simulink model "et_robocon_dev_guy"  (R2013b)
settings: Solver=FixedStepDiscrete  SolverMode=SingleTasking  StartTime=0.0  StopTime=inf  FixedStep=balancer_ts  RelTol=1e-3
undefined symbols (not defined in the file): a_d, a_r, balancerStates_Bus0, Batt, battery_gain, battery_offset, cmd_max, current_mode_status, current_task_operation_status, DiscIntNeverNeededParam, exec_period, Init_Bus0, k_f, k_i, k_phidot, k_thetadot, lightCalib, R, STATE, TRACK_MODE_LIST, ts2, W
libraries: simulink x29, legonxtlib x28, simulink_extras x4, light_sensor_calibration_algorithm_atomic_sub_chart_library x3, gyro_calibration_algorithm_atomic_sub_chart_library x1, limbo_algorithm_atomic_sub_chart_library x1, see_saw x1
(part 2 of 3)

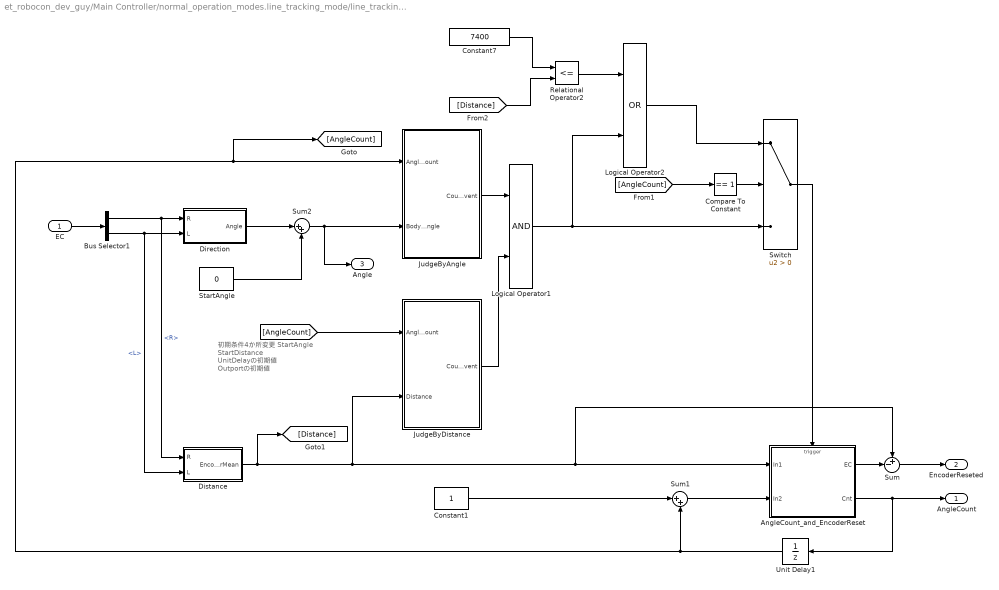
== system et_robocon_dev_guy/Main Controller/normal_operation_modes.line_tracking_mode/line_tracking_mode.processLight/LineTracePID/AngleCounter ==
  note: 初期条件4か所変更
      | StartAngle
      | StartDistance
      | UnitDelayの初期値
      | Outportの初期値
  EC : Inport
  AngleCount_and_EncoderReset : Subsystem  TreatAsAtomicUnit=on
  Bus Selector1 : BusSelector  OutputSignals=R,L
  Compare To Constant : simulink/Logic and Bit Operations/Compare To Constant  relop===  const=1  OutDataTypeStr=boolean
  Constant1 : Constant  OutDataTypeStr=uint8
  Constant7 : Constant  Value=7400  OutDataTypeStr=int32
  Direction : Subsystem
  Distance : Subsystem
  JudgeByAngle : Subsystem
  JudgeByDistance : Subsystem
  Logical Operator1 : Logic  AllPortsSameDT=off  OutDataTypeStr=boolean
  Logical Operator2 : Logic  Operator=OR  AllPortsSameDT=off  OutDataTypeStr=boolean
  Relational Operator2 : RelationalOperator  Operator=<=  OutDataTypeStr=boolean
  StartAngle : Constant  Value=0  OutDataTypeStr=int16
  Sum : Sum  Inputs=+-|
  Sum1 : Sum  Inputs=|++  AccumDataTypeStr=uint8
  Sum2 : Sum  Inputs=|++
  Switch : Switch  Criteria=u2 > Threshold
  Unit Delay1 : UnitDelay  InitialCondition=1  SampleTime=-1
  AngleCount : Outport
  EncoderReseted : Outport  Port=2
  Angle : Outport  Port=3
  wires:
  Sum2/1 -> JudgeByAngle/2(BodyAngle), Angle/1
  Sum1/1 -> AngleCount_and_EncoderReset/2(In2)
  Constant1/1 -> Sum1/1
  Unit Delay1/1 -> [AngleCount], JudgeByAngle/1(AngleCount), Sum1/2
  AngleCount_and_EncoderReset/2(Cnt) -> AngleCount/1, Unit Delay1/1
  Bus Selector1/1 -> Distance/1(R), Direction/1(R)  "<R>"
  Bus Selector1/2 -> Distance/2(L), Direction/2(L)  "<L>"
  EC/1 -> Bus Selector1/1
  AngleCount_and_EncoderReset/1(EC) -> Sum/2
  Sum/1 -> EncoderReseted/1
  Distance/1(EncoderMean) -> [Distance], JudgeByDistance/2(Distance), Sum/1, AngleCount_and_EncoderReset/1(In1)
  [AngleCount] -> JudgeByDistance/1(AngleCount)
  JudgeByAngle/1(CountEvent) -> Logical Operator1/1
  JudgeByDistance/1(CountEvent) -> Logical Operator1/2
  Direction/1(Angle) -> Sum2/1
  StartAngle/1 -> Sum2/2
  Logical Operator1/1 -> Logical Operator2/2, Switch/3
  Switch/1 -> AngleCount_and_EncoderReset/Trigger
  Compare To Constant/1 -> Switch/2
  [AngleCount] -> Compare To Constant/1
  Logical Operator2/1 -> Switch/1
  Constant7/1 -> Relational Operator2/1
  Relational Operator2/1 -> Logical Operator2/1
  [Distance] -> Relational Operator2/2

== system et_robocon_dev_guy/Main Controller/normal_operation_modes.line_tracking_mode/line_tracking_mode.processLight/LineTracePID/Handler ==
  steering : Inport
  fwd : Inport  Port=2
  sw : Inport  Port=3
  Constant1 : Constant  Value=-1  OutDataTypeStr=int8
  Lookup Table : Lookup  InputValues="[-30  -5  0  5 30]"  Table=[0.65 1 1 1 0.65]  RndMeth=Simplest
  Mux : Mux  Inputs=2
  Product : Product  OutDataTypeStr=single  RndMeth=Simplest
  Switch : Switch  OutDataTypeStr=single  RndMeth=Simplest
  Switch1 : Switch  OutDataTypeStr=single  RndMeth=Simplest
  rocket_start : Subsystem
  slow_start : Subsystem
  Out1 : Outport
  wires:
  Lookup Table/1 -> Product/2
  Product/1 -> Switch/3
  fwd/1 -> Switch/1, Product/1
  steering/1 -> Lookup Table/1, Mux/2  "str"
  sw/1 -> Switch/2
  slow_start/1(fwd_slow) -> Switch1/1
  Mux/1 -> Out1/1
  Switch/1 -> rocket_start/1(fwd), slow_start/1(fwd)  "fwd"
  Constant1/1 -> Switch1/2
  rocket_start/1(fwd_slow) -> Switch1/3
  Switch1/1 -> Mux/1

== system et_robocon_dev_guy/Main Controller/normal_operation_modes.line_tracking_mode/line_tracking_mode.processLight/LineTracePID/SwitchController ==
  Cnt : Inport
  EC_reseted : Inport  Port=2
  Angle : Inport  Port=3
  LigthSens : Inport  Port=4
  Gyro : Inport  Port=5
  BasicStage : Subsystem
  BonusStage : Subsystem
  Merge : Merge
  Merge1 : Merge
  Merge2 : Merge
  Flag_steering : Outport
  PID : Outport  Port=2
  fwd : Outport  Port=3
  bias : Outport  Port=4
  wires:
  Cnt/1 -> BonusStage/1(AngleCnt), BasicStage/1(AngleCnt)
  Merge/1 -> PID/1
  Merge1/1 -> fwd/1
  BasicStage/2(fwd) -> [fwd_Basic]
  [fwd_Basic] -> Merge1/1
  [fwd_Bonus] -> Merge1/2
  BasicStage/4(bias) -> [bias_Basic]
  [bias_Basic] -> Merge2/1
  [bias_Bonus] -> Merge2/2
  Merge2/1 -> bias/1
  EC_reseted/1 -> BasicStage/2(EC_reseted), BonusStage/2(EC_reseted)
  LigthSens/1 -> BonusStage/4(LightSens), BasicStage/4(LightSens)
  BasicStage/1(PID) -> Merge/1
  Gyro/1 -> BonusStage/3(Gyro)
  BonusStage/1(PID) -> Merge/2
  BonusStage/2(fwd) -> [fwd_Bonus]
  BonusStage/3(bias) -> [bias_Bonus]
  Angle/1 -> BasicStage/3(Angle)
  BasicStage/3(Flag_steering) -> Flag_steering/1

== system et_robocon_dev_guy/Main Controller/normal_operation_modes.line_tracking_mode/line_tracking_mode.processLight/LineTracePID/SwutchForFreeSteering ==
  note: Edge Change
      | -1: Run right edge
      | 1: Run left edge
  note: Target Value
  FlagSteering : Inport
  PID : Inport  Port=2
  LightSens : Inport  Port=3
  Add : Sum  Inputs=+-  AccumDataTypeStr=single  OutDataTypeStr=single  RndMeth=Simplest
  AdjustForUnit : Gain  Gain=18.25  OutDataTypeStr=single  RndMeth=Simplest
  Constant2 : Constant  OutDataTypeStr=single  SampleTime=-1
  Constant6 : Constant  Value=0.5  OutDataTypeStr=single  SampleTime=-1
  DeleteDummyData : Selector  InputPortWidth=5  IndexOptions=Index vector (dialog)  Indices=1  OutputSizes=1
  Product1 : Product  OutDataTypeStr=single  RndMeth=Simplest
  Switch : Switch  Criteria=u2 > Threshold
  tmpController : Subsystem  TreatAsAtomicUnit=on  mask(tmp PID Controller){Ts_=ts2, SaturationMax=100, SaturationMin=-100}
      mask prompts: Ts_ "Sampling Time (Task Period)"; SaturationMax "Saturation Max Value of PID Ctrl"; SaturationMin "Saturation Min Value of PID"
      mask help:
      | Sampling Time: Task Period
      | P: Proportional Gain
      | I: Integral Gain
      | D: Derivative Gain
      | B: Back Gain for Integrator
      | Saturation Max Value of PID ctrl:
      |    Saturation Max Value of PID ctrl > Saturation Min Value of PID ctrl
      | Saturation Min Value of PID ctrl:
      |    Saturation Min Value of PID ctrl < Saturation Max Value of PID ctrl
      settings: RTWSystemCode=Inline
      mask Display: disp('PID')
  Steering : Outport
  wires:
  PID/1 -> tmpController/2(BD), DeleteDummyData/1
  Switch/1 -> Steering/1
  DeleteDummyData/1 -> Switch/1  "FreeSteering"
  FlagSteering/1 -> Switch/2
  Add/1 -> Product1/1
  LightSens/1 -> Add/1
  Constant6/1 -> Add/2
  Constant2/1 -> Product1/2
  Product1/1 -> tmpController/1(Error)  "Diff_Between_Target_and_Value"
  tmpController/1(Target_deg) -> AdjustForUnit/1
  AdjustForUnit/1 -> Switch/3  "LintTraceSteering"

== system et_robocon_dev_guy/State Estimation/Data Type Conversion Unit Conversion Tail Initialization/Low Pass Filter/Store Offset ==
  x : Inport
  Enable : EnablePort
  x0 : Outport  InitialOutput=0
  wires:
  x/1 -> x0/1

== system et_robocon_dev_guy/State Estimation/Data Type Conversion Unit Conversion Tail Initialization/tail processing/tail initialization ==
  tail : Inport
  Trigger : TriggerPort  PortDimensions=1
  tail_0 : Outport  InitialOutput=0
  wires:
  tail/1 -> tail_0/1

== system et_robocon_dev_guy/State Estimation/Gyro Processing/Compute psi/Very Low Pass Filter ==
  In1 : Inport
  Gain2 : Gain  Gain=0.004
  Gain3 : Gain  Gain=0.996
  Sum2 : Sum  Inputs=|++
  Unit Delay External IC : simulink/Additional Math & Discrete/Additional Discrete/Unit Delay External IC  tsamp=-1
  Out1 : Outport
  wires:
  Gain3/1 -> Sum2/2
  Sum2/1 -> Out1/1, Unit Delay External IC/1
  Gain2/1 -> Sum2/1
  Unit Delay External IC/1 -> Gain3/1
  In1/1 -> Gain2/1, Unit Delay External IC/2

== system et_robocon_dev_guy/State Estimation/StateEstimation/Process theta1/Enabled Subsystem ==
  x : Inport
  Enable : EnablePort
  x0 : Outport  InitialOutput=0
  wires:
  x/1 -> x0/1

== system et_robocon_dev_guy/State Estimation/StateEstimation/Process theta1/LPF and deriv ==
  theta : Inport
  Gain : Gain  Gain=1/0.004
  Low Pass Filter : DiscreteFilter  Numerator=[.2]  Denominator=[1 -0.8]
  Sum3 : Sum  Inputs=+-
  Unit Delay : UnitDelay  SampleTime=-1
  theta_dot : Outport
  wires:
  Unit Delay/1 -> Sum3/2
  Gain/1 -> Unit Delay/1, Sum3/1
  Sum3/1 -> theta_dot/1  "theta_dot"
  Low Pass Filter/1 -> Gain/1
  theta/1 -> Low Pass Filter/1

== system et_robocon_dev_guy/State Estimation/StateEstimation/Process theta1/LPF and deriv1 ==
  theta_dot : Inport
  Gain : Gain  Gain=1/0.004
  Low Pass Filter : DiscreteFilter  Numerator=[.2]  Denominator=[1 -0.8]
  Sum3 : Sum  Inputs=+-
  Unit Delay : UnitDelay  SampleTime=-1
  theta_dot_dot : Outport
  wires:
  theta_dot/1 -> Low Pass Filter/1
  Low Pass Filter/1 -> Gain/1
  Sum3/1 -> theta_dot_dot/1  "theta_dot_dot"
  Gain/1 -> Sum3/1, Unit Delay/1
  Unit Delay/1 -> Sum3/2

== system et_robocon_dev_guy/State Estimation/StateEstimation/Process theta1/Store x0 ==
  x : Inport
  Enable : EnablePort
  x0 : Outport  InitialOutput=0
  wires:
  x/1 -> x0/1

== system et_robocon_dev_guy/Main Controller/normal_operation_modes.line_tracking_mode/line_tracking_mode.balanceControl/ForSimulation/Cal_PWM/Cal_vol_max ==
  battery : Inport
  Constant : Constant  Value=battery_offset  OutDataTypeStr=single  SampleTime=-1
      settings: AttributesFormatString=DataType = %<OutDataTypeStr>
  Gain3 : Gain  Gain=battery_gain  OutDataTypeStr=Inherit: Same as input  ParamDataTypeStr=Inherit: Same as input
  Sum2 : Sum  Inputs=|+-  OutDataTypeStr=Inherit: Same as first input
  vol_max : Outport
  wires:
  Constant/1 -> Sum2/2
  Sum2/1 -> vol_max/1  "base_pwm"
  Gain3/1 -> Sum2/1
  battery/1 -> Gain3/1

== system et_robocon_dev_guy/Main Controller/normal_operation_modes.line_tracking_mode/line_tracking_mode.balanceControl/ForSimulation/Cal_Reference/DiscreteIntegrator ==
  in : Inport
  Gain : Gain  Gain=exec_period  OutDataTypeStr=Inherit: Same as input  ParamDataTypeStr=Inherit: Same as input
  Sum : Sum  Inputs=|++  OutDataTypeStr=Inherit: Same as first input
  Unit Delay : UnitDelay  SampleTime=-1  StateName=ud_theta_ref  StateMustResolveToSignalObject=on
      settings: AttributesFormatString=Signal name = ud_theta_ref
  out : Outport
  wires:
  Unit Delay/1 -> Sum/2, out/1
  Gain/1 -> Sum/1
  Sum/1 -> Unit Delay/1
  in/1 -> Gain/1

== system et_robocon_dev_guy/Main Controller/normal_operation_modes.line_tracking_mode/line_tracking_mode.balanceControl/ForSimulation/Cal_Reference/LowPathFilter ==
  note: Low Path Filter Function
      |               1-a_r
      |          ----------------
      |          1-a_r*z^(-1)
  in : Inport
  Constant : Constant  OutDataTypeStr=single
      settings: AttributesFormatString=DataType = %<OutDataTypeStr>
  Constant1 : Constant  Value=a_r  OutDataTypeStr=single
      settings: AttributesFormatString=DataType = %<OutDataTypeStr>
  Gain2 : Gain  Gain=a_r  OutDataTypeStr=Inherit: Same as input  ParamDataTypeStr=Inherit: Same as input
  Product : Product  RndMeth=Zero
  Sum : Sum  Inputs=|++  OutDataTypeStr=Inherit: Same as first input
  Sum1 : Sum  Inputs=|+-
  Unit Delay : UnitDelay  SampleTime=-1  StateName=ud_thetadot_cmd_lpf  StateMustResolveToSignalObject=on
      settings: AttributesFormatString=Signal name = ud_thetadot_cmd_lpf
  out : Outport
  wires:
  Sum/1 -> Unit Delay/1, out/1
  Unit Delay/1 -> Gain2/1
  Gain2/1 -> Sum/2
  Product/1 -> Sum/1
  in/1 -> Product/1
  Constant/1 -> Sum1/1
  Sum1/1 -> Product/2
  Constant1/1 -> Sum1/2

== system et_robocon_dev_guy/Main Controller/normal_operation_modes.line_tracking_mode/line_tracking_mode.balanceControl/ForSimulation/Cal_x1/DiscreteDerivative ==
  in : Inport
  in1 : Inport  Port=2
  Constant : Constant  Value=exec_period  OutDataTypeStr=single
  Product : Product  Inputs=*/  RndMeth=Simplest
  Sum : Sum  Inputs=|+-  OutDataTypeStr=Inherit: Same as first input
  out : Outport
  wires:
  Sum/1 -> Product/1
  in1/1 -> Sum/2
  in/1 -> Sum/1
  Product/1 -> out/1
  Constant/1 -> Product/2

== system et_robocon_dev_guy/Main Controller/normal_operation_modes.line_tracking_mode/line_tracking_mode.balanceControl/ForSimulation/Cal_x1/DiscreteIntegrator ==
  in : Inport
  Gain : Gain  Gain=exec_period  OutDataTypeStr=Inherit: Same as input  ParamDataTypeStr=Inherit: Same as input
  Sum : Sum  Inputs=|++  OutDataTypeStr=Inherit: Same as first input
  Unit Delay : UnitDelay  SampleTime=-1
      settings: AttributesFormatString=Signal name = ud_psi
  out : Outport
  wires:
  Unit Delay/1 -> Sum/2, out/1
  Gain/1 -> Sum/1
  Sum/1 -> Unit Delay/1
  in/1 -> Gain/1

== system et_robocon_dev_guy/Main Controller/normal_operation_modes.line_tracking_mode/line_tracking_mode.balanceControl/ForSimulation/Cal_x1/LowPathFilter ==
  note: Low Path Filter Function
      |               1-a_d
      |          ----------------
      |          1-a_d*z^(-1)
  in : Inport
  Constant : Constant  OutDataTypeStr=single
      settings: AttributesFormatString=DataType = %<OutDataTypeStr>
  Constant1 : Constant  Value=a_d  OutDataTypeStr=single
      settings: AttributesFormatString=DataType = %<OutDataTypeStr>
  Gain2 : Gain  Gain=a_d  OutDataTypeStr=Inherit: Same as input  ParamDataTypeStr=Inherit: Same as input
  Product : Product  RndMeth=Zero
  Sum : Sum  Inputs=|++  OutDataTypeStr=Inherit: Same as first input
  Sum1 : Sum  Inputs=|+-
  Unit Delay : UnitDelay  SampleTime=-1  StateName=ud_theta_lpf  StateMustResolveToSignalObject=on
      settings: AttributesFormatString=Signal name = ud_thta_lpf
  out : Outport
  out1 : Outport  Port=2
  wires:
  Constant1/1 -> Sum1/2
  Sum1/1 -> Product/2
  Constant/1 -> Sum1/1
  in/1 -> Product/1
  Product/1 -> Sum/1
  Gain2/1 -> Sum/2
  Unit Delay/1 -> Gain2/1, out1/1
  Sum/1 -> out/1, Unit Delay/1  "theta_lpf"

== system et_robocon_dev_guy/Main Controller/normal_operation_modes.line_tracking_mode/line_tracking_mode.processLight/LineTracePID/AngleCounter/AngleCount_and_EncoderReset ==
  In1 : Inport
  In2 : Inport  Port=2  OutDataTypeStr=uint8
  Trigger : TriggerPort
  Data Store Read : DataStoreRead  DataStoreName=fwd_premode_last
  Data Store Write : DataStoreWrite  DataStoreName=fwd_postmode_init
  EC : Outport
  Cnt : Outport  Port=2  InitialOutput=1
  wires:
  In2/1 -> Cnt/1
  In1/1 -> EC/1
  Data Store Read/1 -> Data Store Write/1

== system et_robocon_dev_guy/Main Controller/normal_operation_modes.line_tracking_mode/line_tracking_mode.processLight/LineTracePID/AngleCounter/Direction ==
  note: 160: Distance between left tire and right tire
      | 41: Radius of tire
  R : Inport
  L : Inport  Port=2
  Gain2 : Gain  Gain=41/160
  Subtract1 : Sum  Inputs=+-
  Angle : Outport
  wires:
  Gain2/1 -> Angle/1
  R/1 -> Subtract1/1
  L/1 -> Subtract1/2
  Subtract1/1 -> Gain2/1

== system et_robocon_dev_guy/Main Controller/normal_operation_modes.line_tracking_mode/line_tracking_mode.processLight/LineTracePID/AngleCounter/Distance ==
  R : Inport
  L : Inport  Port=2
  Gain1 : Gain  Gain=1/2
  Subtract : Sum
  EncoderMean : Outport
  wires:
  Gain1/1 -> EncoderMean/1
  Subtract/1 -> Gain1/1
  L/1 -> Subtract/2
  R/1 -> Subtract/1

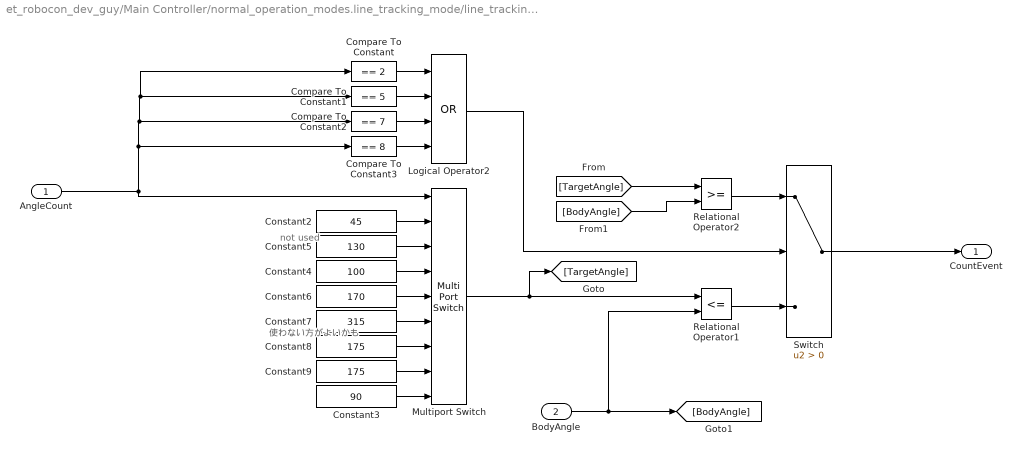
== system et_robocon_dev_guy/Main Controller/normal_operation_modes.line_tracking_mode/line_tracking_mode.processLight/LineTracePID/AngleCounter/JudgeByAngle ==
  note: not used
  note: 使わない方がよいかも
  AngleCount : Inport
  BodyAngle : Inport  Port=2
  Compare To Constant : simulink/Logic and Bit Operations/Compare To Constant  relop===  const=2  OutDataTypeStr=boolean
  Compare To Constant1 : simulink/Logic and Bit Operations/Compare To Constant  relop===  const=5  OutDataTypeStr=boolean
  Compare To Constant2 : simulink/Logic and Bit Operations/Compare To Constant  relop===  const=7  OutDataTypeStr=boolean
  Compare To Constant3 : simulink/Logic and Bit Operations/Compare To Constant  relop===  const=8  OutDataTypeStr=boolean
  Constant2 : Constant  Value=45  OutDataTypeStr=int32
  Constant3 : Constant  Value=90  OutDataTypeStr=int32
  Constant4 : Constant  Value=100  OutDataTypeStr=int32
  Constant5 : Constant  Value=130  OutDataTypeStr=int32
  Constant6 : Constant  Value=170  OutDataTypeStr=int32
  Constant7 : Constant  Value=315  OutDataTypeStr=int32
  Constant8 : Constant  Value=175  OutDataTypeStr=int32
  Constant9 : Constant  Value=175  OutDataTypeStr=int32
  Logical Operator2 : Logic  Operator=OR  Inputs=4  AllPortsSameDT=off  OutDataTypeStr=boolean
  Multiport Switch : MultiPortSwitch  Inputs=8  DiagnosticForDefault=None
  Relational Operator1 : RelationalOperator  Operator=<=  OutDataTypeStr=boolean
  Relational Operator2 : RelationalOperator  OutDataTypeStr=boolean
  Switch : Switch  Criteria=u2 > Threshold
  CountEvent : Outport
  wires:
  Constant3/1 -> Multiport Switch/9
  Relational Operator1/1 -> Switch/3
  Compare To Constant2/1 -> Logical Operator2/3
  Compare To Constant3/1 -> Logical Operator2/4
  Compare To Constant1/1 -> Logical Operator2/2
  Compare To Constant/1 -> Logical Operator2/1
  Relational Operator2/1 -> Switch/1
  Logical Operator2/1 -> Switch/2
  AngleCount/1 -> Compare To Constant/1, Compare To Constant1/1, Compare To Constant2/1, Compare To Constant3/1, Multiport Switch/1
  BodyAngle/1 -> [BodyAngle], Relational Operator1/2
  Constant9/1 -> Multiport Switch/8
  Multiport Switch/1 -> [TargetAngle], Relational Operator1/1
  Constant4/1 -> Multiport Switch/4
  Constant8/1 -> Multiport Switch/7
  Constant5/1 -> Multiport Switch/3
  Constant2/1 -> Multiport Switch/2
  Constant6/1 -> Multiport Switch/5
  Constant7/1 -> Multiport Switch/6
  [BodyAngle] -> Relational Operator2/2
  [TargetAngle] -> Relational Operator2/1
  Switch/1 -> CountEvent/1

== system et_robocon_dev_guy/Main Controller/normal_operation_modes.line_tracking_mode/line_tracking_mode.processLight/LineTracePID/AngleCounter/JudgeByDistance ==
  AngleCount : Inport
  Distance : Inport  Port=2
  Constant1 : Constant  Value=14700  OutDataTypeStr=int32
  Constant10 : Constant  Value=9700  OutDataTypeStr=int32
  Constant2 : Constant  Value=7200  OutDataTypeStr=int32
  Constant3 : Constant  Value=18700  OutDataTypeStr=int32
  Constant4 : Constant  Value=11550  OutDataTypeStr=int32
  Constant5 : Constant  Value=9950  OutDataTypeStr=int32
  Constant6 : Constant  Value=12000  OutDataTypeStr=int32
  Constant7 : Constant  Value=11800  OutDataTypeStr=int32
  Constant8 : Constant  Value=17100  OutDataTypeStr=int32
  Constant9 : Constant  Value=17800  OutDataTypeStr=int32
  Multiport Switch : MultiPortSwitch  Inputs=8  DiagnosticForDefault=None
  Relational Operator2 : RelationalOperator  Operator=<=  OutDataTypeStr=boolean
  StartDistance : Constant  Value=0  OutDataTypeStr=int32
  Sum2 : Sum  Inputs=|+-
  Terminator : Terminator
  Terminator1 : Terminator
  CountEvent : Outport
  wires:
  Constant1/1 -> Multiport Switch/6
  Constant6/1 -> Multiport Switch/5
  Constant2/1 -> Multiport Switch/2
  Constant5/1 -> Multiport Switch/3
  Constant8/1 -> Multiport Switch/7
  Constant4/1 -> Multiport Switch/4
  Constant9/1 -> Multiport Switch/8
  Distance/1 -> Relational Operator2/2
  Constant3/1 -> Multiport Switch/9
  Multiport Switch/1 -> Sum2/1
  StartDistance/1 -> Sum2/2
  Sum2/1 -> Relational Operator2/1
  Relational Operator2/1 -> CountEvent/1
  AngleCount/1 -> Multiport Switch/1
  Constant7/1 -> Terminator/1
  Constant10/1 -> Terminator1/1

== system et_robocon_dev_guy/Main Controller/normal_operation_modes.line_tracking_mode/line_tracking_mode.processLight/LineTracePID/Handler/rocket_start ==
  fwd : Inport
  Constant : Constant  Value=2  OutDataTypeStr=single  SampleTime=-1
  Saturation : Saturate  UpperLimit=200  LowerLimit=0  RndMeth=Simplest
  Sum : Sum  Inputs=|++  AccumDataTypeStr=single  OutDataTypeStr=single  RndMeth=Simplest  InputSameDT=on
  Sum1 : Sum  Inputs=-+  AccumDataTypeStr=single  OutDataTypeStr=single  RndMeth=Simplest
  Switch : Switch  Criteria=u2 > Threshold  OutDataTypeStr=single  RndMeth=Simplest
  Unit Delay1 : UnitDelay  InitialCondition=100  SampleTime=-1
  fwd_slow : Outport
  wires:
  Saturation/1 -> Switch/3, Sum1/2
  fwd/1 -> Switch/1, Sum1/1
  Switch/1 -> fwd_slow/1
  Sum1/1 -> Switch/2
  Sum/1 -> Saturation/1, Unit Delay1/1
  Constant/1 -> Sum/1
  Unit Delay1/1 -> Sum/2

== system et_robocon_dev_guy/Main Controller/normal_operation_modes.line_tracking_mode/line_tracking_mode.processLight/LineTracePID/Handler/slow_start ==
  fwd : Inport
  Constant : Constant  Value=2  OutDataTypeStr=single  SampleTime=-1
  Saturation : Saturate  UpperLimit=200  LowerLimit=0  RndMeth=Simplest
  Sum : Sum  Inputs=|++  AccumDataTypeStr=single  OutDataTypeStr=single  RndMeth=Simplest  InputSameDT=on
  Sum1 : Sum  Inputs=-+  AccumDataTypeStr=single  OutDataTypeStr=single  RndMeth=Simplest
  Switch : Switch  Criteria=u2 > Threshold  OutDataTypeStr=single  RndMeth=Simplest
  Unit Delay1 : UnitDelay  InitialCondition=30  SampleTime=-1
  fwd_slow : Outport
  wires:
  Saturation/1 -> Switch/3, Sum1/2
  fwd/1 -> Switch/1, Sum1/1
  Switch/1 -> fwd_slow/1
  Sum1/1 -> Switch/2
  Sum/1 -> Saturation/1, Unit Delay1/1
  Constant/1 -> Sum/1
  Unit Delay1/1 -> Sum/2

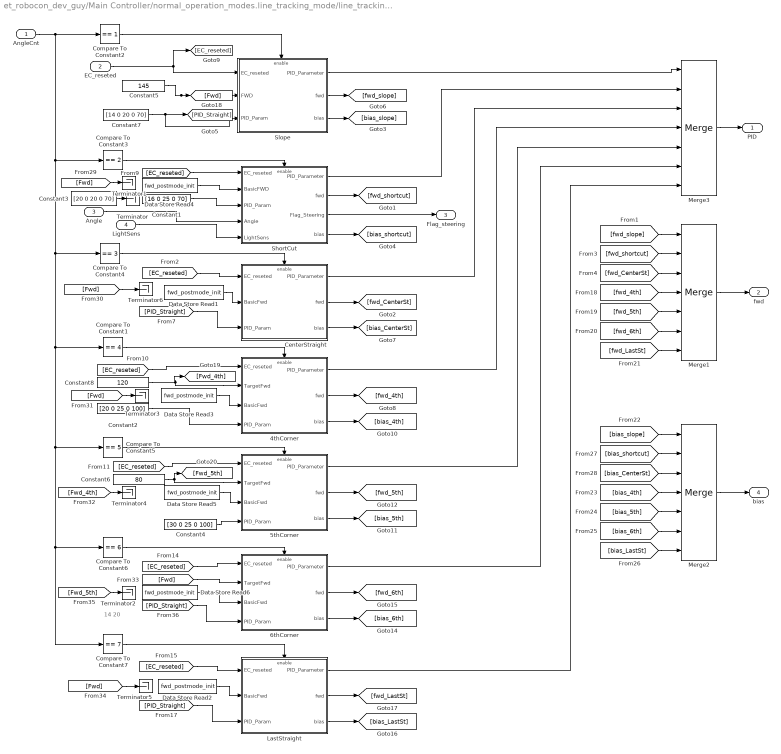
== system et_robocon_dev_guy/Main Controller/normal_operation_modes.line_tracking_mode/line_tracking_mode.processLight/LineTracePID/SwitchController/BasicStage ==
  note: 14 20
  AngleCnt : Inport
  EC_reseted : Inport  Port=2
  Angle : Inport  Port=3
  LightSens : Inport  Port=4
  4thCorner : Subsystem  TreatAsAtomicUnit=on
  5thCorner : Subsystem  TreatAsAtomicUnit=on
  6thCorner : Subsystem  TreatAsAtomicUnit=on
  CenterStraight : Subsystem  TreatAsAtomicUnit=on
  Compare To Constant1 : simulink/Logic and Bit Operations/Compare To Constant  relop===  const=4  OutDataTypeStr=uint8
  Compare To Constant2 : simulink/Logic and Bit Operations/Compare To Constant  relop===  const=1  OutDataTypeStr=uint8
  Compare To Constant3 : simulink/Logic and Bit Operations/Compare To Constant  relop===  const=2  OutDataTypeStr=uint8
  Compare To Constant4 : simulink/Logic and Bit Operations/Compare To Constant  relop===  const=3  OutDataTypeStr=uint8
  Compare To Constant5 : simulink/Logic and Bit Operations/Compare To Constant  relop===  const=5  OutDataTypeStr=uint8
  Compare To Constant6 : simulink/Logic and Bit Operations/Compare To Constant  relop===  const=6  OutDataTypeStr=uint8
  Compare To Constant7 : simulink/Logic and Bit Operations/Compare To Constant  relop===  const=7  OutDataTypeStr=uint8
  Constant1 : Constant  Value=[16 0 25 0 70]  OutDataTypeStr=single  SampleTime=-1
  Constant2 : Constant  Value=[20 0 25 0 100]  OutDataTypeStr=single  SampleTime=-1
  Constant3 : Constant  Value=[20 0 20 0 70]  OutDataTypeStr=single  SampleTime=-1
  Constant4 : Constant  Value=[30 0 25 0 100]  OutDataTypeStr=single  SampleTime=-1
  Constant5 : Constant  Value=145  OutDataTypeStr=single  SampleTime=-1
  Constant6 : Constant  Value=80  OutDataTypeStr=single  SampleTime=-1
  Constant7 : Constant  Value=[14 0 20 0 70]  OutDataTypeStr=single  SampleTime=-1
  Constant8 : Constant  Value=120  OutDataTypeStr=single  SampleTime=-1
  Data Store Read{1..6} (6 alike) : DataStoreRead  DataStoreName=fwd_postmode_init
  LastStraight : Subsystem  TreatAsAtomicUnit=on
  Merge1 : Merge  Inputs=7
  Merge2 : Merge  Inputs=7
  Merge3 : Merge  Inputs=7
  ShortCut : Subsystem  TreatAsAtomicUnit=on
  Slope : Subsystem  TreatAsAtomicUnit=on
  Terminator{,1..6} (7 alike) : Terminator
  PID : Outport
  fwd : Outport  Port=2
  Flag_steering : Outport  Port=3
  bias : Outport  Port=4
  wires:
  AngleCnt/1 -> Compare To Constant2/1, Compare To Constant7/1, Compare To Constant6/1, Compare To Constant5/1, Compare To Constant1/1, Compare To Constant4/1, Compare To Constant3/1
  Compare To Constant2/1 -> Slope/Enable
  Merge1/1 -> fwd/1
  Compare To Constant3/1 -> ShortCut/Enable
  Compare To Constant4/1 -> CenterStraight/Enable
  [fwd_slope] -> Merge1/1
  [fwd_shortcut] -> Merge1/2
  [fwd_CenterSt] -> Merge1/3
  Constant7/1 -> Slope/3(PID_Param), [PID_Straight]
  [EC_reseted] -> ShortCut/1(EC_reseted)
  [EC_reseted] -> CenterStraight/1(EC_reseted)
  Compare To Constant1/1 -> 4thCorner/Enable
  Compare To Constant5/1 -> 5thCorner/Enable
  Compare To Constant6/1 -> 6thCorner/Enable
  Compare To Constant7/1 -> LastStraight/Enable
  EC_reseted/1 -> Slope/1(EC_reseted), [EC_reseted]
  [EC_reseted] -> 4thCorner/1(EC_reseted)
  [EC_reseted] -> 5thCorner/1(EC_reseted)
  [EC_reseted] -> 6thCorner/1(EC_reseted)
  [EC_reseted] -> LastStraight/1(EC_reseted)
  [fwd_4th] -> Merge1/4
  [fwd_5th] -> Merge1/5
  [fwd_LastSt] -> Merge1/7
  [fwd_6th] -> Merge1/6
  [bias_slope] -> Merge2/1
  [bias_shortcut] -> Merge2/2
  [bias_CenterSt] -> Merge2/3
  [bias_4th] -> Merge2/4
  [bias_5th] -> Merge2/5
  [bias_LastSt] -> Merge2/7
  [bias_6th] -> Merge2/6
  Slope/2(fwd) -> [fwd_slope]
  ShortCut/2(fwd) -> [fwd_shortcut]
  CenterStraight/2(fwd) -> [fwd_CenterSt]
  4thCorner/2(fwd) -> [fwd_4th]
  5thCorner/2(fwd) -> [fwd_5th]
  6thCorner/2(fwd) -> [fwd_6th]
  LastStraight/2(fwd) -> [fwd_LastSt]
  Merge3/1 -> PID/1
  Merge2/1 -> bias/1
  LastStraight/3(bias) -> [bias_LastSt]
  6thCorner/3(bias) -> [bias_6th]
  5thCorner/3(bias) -> [bias_5th]
  Slope/1(PID_Parameter) -> Merge3/1
  Slope/3(bias) -> [bias_slope]
  ShortCut/1(PID_Parameter) -> Merge3/2
  ShortCut/4(bias) -> [bias_shortcut]
  CenterStraight/1(PID_Parameter) -> Merge3/3
  CenterStraight/3(bias) -> [bias_CenterSt]
  4thCorner/1(PID_Parameter) -> Merge3/4
  4thCorner/3(bias) -> [bias_4th]
  5thCorner/1(PID_Parameter) -> Merge3/5
  6thCorner/1(PID_Parameter) -> Merge3/6
  LastStraight/1(PID_Parameter) -> Merge3/7
  Constant1/1 -> ShortCut/3(PID_Param)
  Angle/1 -> ShortCut/4(Angle)
  [PID_Straight] -> LastStraight/3(PID_Param)
  [PID_Straight] -> 6thCorner/4(PID_Param)
  Constant4/1 -> 5thCorner/4(PID_Param)
  Constant2/1 -> 4thCorner/4(PID_Param)
  [PID_Straight] -> CenterStraight/3(PID_Param)
  LightSens/1 -> ShortCut/5(LightSens)
  ShortCut/3(Flag_Steering) -> Flag_steering/1
  Constant5/1 -> Slope/2(FWD), [Fwd]
  [Fwd] -> 6thCorner/2(TargetFwd)
  Constant8/1 -> 4thCorner/2(TargetFwd), [Fwd_4th]
  Constant6/1 -> 5thCorner/2(TargetFwd), [Fwd_5th]
  Constant3/1 -> Terminator/1
  [Fwd] -> Terminator1/1
  Data Store Read4/1 -> ShortCut/2(BasicFWD)
  [Fwd] -> Terminator3/1
  Data Store Read3/1 -> 4thCorner/3(BasicFwd)
  [Fwd_4th] -> Terminator4/1
  Data Store Read5/1 -> 5thCorner/3(BasicFwd)
  [Fwd_5th] -> Terminator2/1
  Data Store Read6/1 -> 6thCorner/3(BasicFwd)
  [Fwd] -> Terminator5/1
  Data Store Read2/1 -> LastStraight/2(BasicFwd)
  [Fwd] -> Terminator6/1
  Data Store Read1/1 -> CenterStraight/2(BasicFwd)

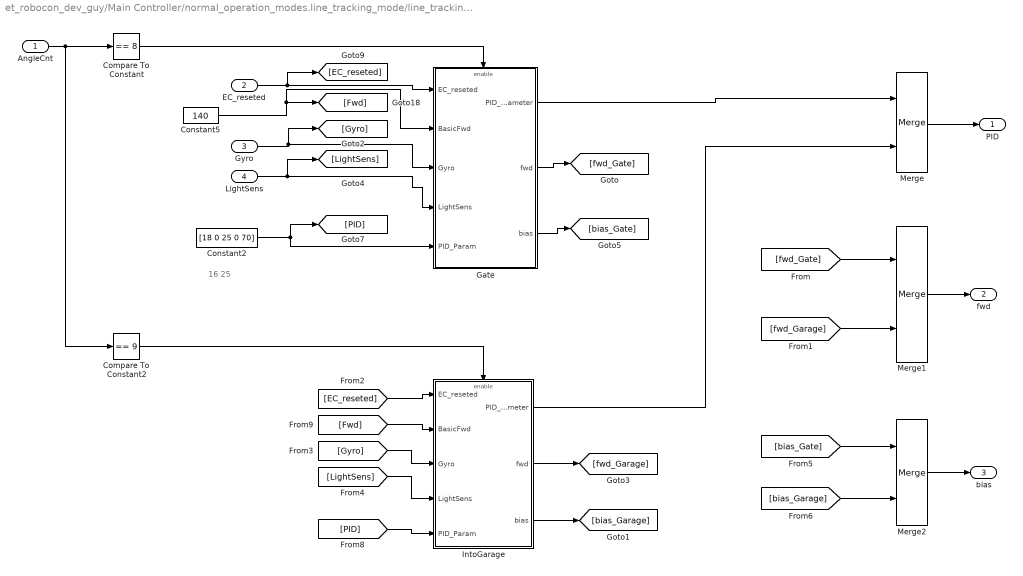
== system et_robocon_dev_guy/Main Controller/normal_operation_modes.line_tracking_mode/line_tracking_mode.processLight/LineTracePID/SwitchController/BonusStage ==
  note: 16 25
  AngleCnt : Inport
  EC_reseted : Inport  Port=2
  Gyro : Inport  Port=3
  LightSens : Inport  Port=4
  Compare To Constant : simulink/Logic and Bit Operations/Compare To Constant  relop===  const=8  OutDataTypeStr=uint8
  Compare To Constant2 : simulink/Logic and Bit Operations/Compare To Constant  relop===  const=9  OutDataTypeStr=uint8
  Constant2 : Constant  Value=[18 0 25 0 70]  OutDataTypeStr=single  SampleTime=-1
  Constant5 : Constant  Value=140  OutDataTypeStr=single  SampleTime=-1
  Gate : Subsystem  TreatAsAtomicUnit=on
  IntoGarage : Subsystem  TreatAsAtomicUnit=on
  Merge : Merge
  Merge1 : Merge
  Merge2 : Merge
  PID : Outport
  fwd : Outport  Port=2
  bias : Outport  Port=3
  wires:
  Compare To Constant/1 -> Gate/Enable
  Compare To Constant2/1 -> IntoGarage/Enable
  EC_reseted/1 -> [EC_reseted], Gate/1(EC_reseted)
  Gate/2(fwd) -> [fwd_Gate]
  Gate/3(bias) -> [bias_Gate]
  LightSens/1 -> [LightSens], Gate/4(LightSens)
  Gyro/1 -> [Gyro], Gate/3(Gyro)
  AngleCnt/1 -> Compare To Constant2/1, Compare To Constant/1
  Merge/1 -> PID/1
  Merge1/1 -> fwd/1
  Merge2/1 -> bias/1
  Gate/1(PID_Parameter) -> Merge/1
  IntoGarage/1(PID_Parameter) -> Merge/2
  [fwd_Garage] -> Merge1/2
  [fwd_Gate] -> Merge1/1
  [bias_Gate] -> Merge2/1
  [bias_Garage] -> Merge2/2
  Constant2/1 -> [PID], Gate/5(PID_Param)
  IntoGarage/2(fwd) -> [fwd_Garage]
  IntoGarage/3(bias) -> [bias_Garage]
  [PID] -> IntoGarage/5(PID_Param)
  [LightSens] -> IntoGarage/4(LightSens)
  [EC_reseted] -> IntoGarage/1(EC_reseted)
  [Gyro] -> IntoGarage/3(Gyro)
  Constant5/1 -> [Fwd], Gate/2(BasicFwd)
  [Fwd] -> IntoGarage/2(BasicFwd)

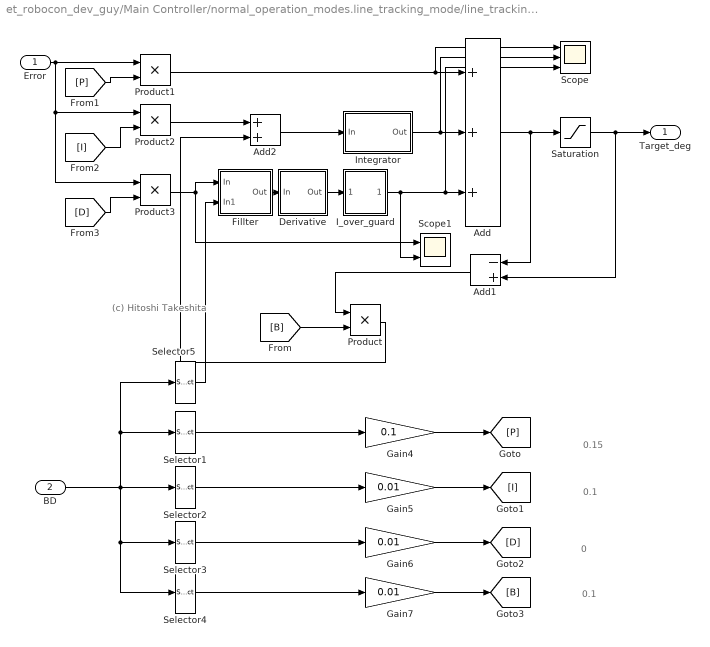
== system et_robocon_dev_guy/Main Controller/normal_operation_modes.line_tracking_mode/line_tracking_mode.processLight/LineTracePID/SwutchForFreeSteering/tmpController ==
  note: (c) Hitoshi Takeshita
  note: 0.15
  note: 0.1
  note: 0
  note: 0.1
  Error : Inport
  BD : Inport  Port=2
  Add : Sum  Inputs=+++  OutDataTypeStr=single  RndMeth=Nearest
  Add1 : Sum  Inputs=-+  OutDataTypeStr=single  RndMeth=Nearest
  Add2 : Sum  OutDataTypeStr=single  RndMeth=Nearest
  Derivative : Subsystem  mask{Ts_=Ts_}
      mask prompts: Ts_ "Sampling Time"
      mask init:
      | Ts_=Ts_;
      mask Display: dpoly([1 -1],[0 Ts_],'z')
  Fillter : Subsystem
  Gain4 : Gain  Gain=0.1
  Gain5 : Gain  Gain=0.01
  Gain6 : Gain  Gain=0.01
  Gain7 : Gain  Gain=0.01
  I_over_guard : Subsystem
  Integrator : Subsystem  mask{Ts_=Ts_}
      mask prompts: Ts_ "Sampling Time"
      mask Display: dpoly([Ts_],[1 -1],'z')
  Product{,1..3} (4 alike) : Product  RndMeth=Zero
  Saturation : Saturate  UpperLimit=SaturationMax  LowerLimit=SaturationMin  LinearizeAsGain=off  OutDataTypeStr=single  RndMeth=Nearest
  Scope : Scope  NumInputPorts=3
      settings: YMin=-5~-5~-5  YMax=5~5~5  SaveName=ScopeData5
  Scope1 : Scope  NumInputPorts=2
      settings: YMin=-5~-5  YMax=5~5  SaveName=ScopeData6
  Selector1 : Selector  InputPortWidth=5  IndexOptions=Index vector (dialog)  Indices=1  OutputSizes=1
  Selector2 : Selector  InputPortWidth=5  IndexOptions=Index vector (dialog)  Indices=2  OutputSizes=1
  Selector3 : Selector  InputPortWidth=5  IndexOptions=Index vector (dialog)  Indices=3  OutputSizes=1
  Selector4 : Selector  InputPortWidth=5  IndexOptions=Index vector (dialog)  Indices=4  OutputSizes=1
  Selector5 : Selector  InputPortWidth=5  IndexOptions=Index vector (dialog)  Indices=5  OutputSizes=1
  Target_deg : Outport
  wires:
  Product/1 -> Add2/2
  Add1/1 -> Product/1
  Add2/1 -> Integrator/1(In)
  Product1/1 -> Add/1, Scope/1
  Integrator/1(Out) -> Add/2, Scope/2
  Add/1 -> Add1/1, Saturation/1
  Derivative/1(Out) -> I_over_guard/1(In1)
  Product2/1 -> Add2/1
  Product3/1 -> Scope1/1, Fillter/1(In)
  Saturation/1 -> Add1/2, Target_deg/1
  Selector1/1 -> Gain4/1
  Selector2/1 -> Gain5/1
  Selector3/1 -> Gain6/1
  Selector4/1 -> Gain7/1
  Gain4/1 -> [P]
  Gain5/1 -> [I]
  Gain6/1 -> [D]
  Gain7/1 -> [B]
  [B] -> Product/2
  [P] -> Product1/2
  [I] -> Product2/2
  [D] -> Product3/2
  BD/1 -> Selector2/1, Selector3/1, Selector4/1, Selector1/1, Selector5/1
  Error/1 -> Product1/1, Product2/1, Product3/1
  I_over_guard/1(Out1) -> Add/3, Scope/3, Scope1/2
  Fillter/1(Out) -> Derivative/1(In)
  Selector5/1 -> Fillter/2(In1)

== system et_robocon_dev_guy/Main Controller/normal_operation_modes.line_tracking_mode/line_tracking_mode.processLight/LineTracePID/SwitchController/BasicStage/4thCorner ==
  EC_reseted : Inport
  TargetFwd : Inport  Port=2
  BasicFwd : Inport  Port=3
  PID_Param : Inport  Port=4
  Enable : EnablePort
  Constant4 : Constant  Value=0
  Normal : Subsystem  TreatAsAtomicUnit=on
  SlowDown : Subsystem
  Speak : Subsystem  TreatAsAtomicUnit=on
  Terminator : Terminator
  Unit Delay : UnitDelay  InitialCondition=1  SampleTime=-1
  PID_Parameter : Outport
  fwd : Outport  Port=2
  bias : Outport  Port=3
  wires:
  PID_Param/1 -> PID_Parameter/1
  Normal/1(Out1) -> bias/1
  Normal/2(fwd) -> fwd/1
  EC_reseted/1 -> Terminator/1
  TargetFwd/1 -> SlowDown/1(TargetFwd)
  BasicFwd/1 -> SlowDown/2(LastFwd)
  SlowDown/1(fwd) -> Normal/1(Fwd)
  Constant4/1 -> Unit Delay/1
  Unit Delay/1 -> Speak/Enable

== system et_robocon_dev_guy/Main Controller/normal_operation_modes.line_tracking_mode/line_tracking_mode.processLight/LineTracePID/SwitchController/BasicStage/5thCorner ==
  EC_reseted : Inport
  TargetFwd : Inport  Port=2
  BasicFwd : Inport  Port=3
  PID_Param : Inport  Port=4
  Enable : EnablePort
  Constant4 : Constant  Value=0
  Normal : Subsystem  TreatAsAtomicUnit=on
  SlowDown : Subsystem
  Speak : Subsystem  TreatAsAtomicUnit=on
  Terminator : Terminator
  Unit Delay : UnitDelay  InitialCondition=1  SampleTime=-1
  PID_Parameter : Outport
  fwd : Outport  Port=2
  bias : Outport  Port=3
  wires:
  EC_reseted/1 -> Terminator/1
  Normal/2(fwd) -> fwd/1
  Normal/1(Out1) -> bias/1
  PID_Param/1 -> PID_Parameter/1
  TargetFwd/1 -> SlowDown/1(TargetFwd)
  BasicFwd/1 -> SlowDown/2(LastFwd)
  SlowDown/1(fwd) -> Normal/1(Fwd)
  Constant4/1 -> Unit Delay/1
  Unit Delay/1 -> Speak/Enable

== system et_robocon_dev_guy/Main Controller/normal_operation_modes.line_tracking_mode/line_tracking_mode.processLight/LineTracePID/SwitchController/BasicStage/6thCorner ==
  EC_reseted : Inport
  TargetFwd : Inport  Port=2
  BasicFwd : Inport  Port=3
  PID_Param : Inport  Port=4
  Enable : EnablePort
  Constant4 : Constant  Value=0
  Normal : Subsystem  TreatAsAtomicUnit=on
  Speak : Subsystem  TreatAsAtomicUnit=on
  SpeedUp : Subsystem
  Terminator : Terminator
  Unit Delay : UnitDelay  InitialCondition=1  SampleTime=-1
  PID_Parameter : Outport
  fwd : Outport  Port=2
  bias : Outport  Port=3
  wires:
  Normal/1(Out1) -> bias/1
  Normal/2(fwd) -> fwd/1
  EC_reseted/1 -> Terminator/1
  BasicFwd/1 -> SpeedUp/2(LastFwd)
  SpeedUp/1(fwd) -> Normal/1(Fwd)
  TargetFwd/1 -> SpeedUp/1(TargetFwd)
  PID_Param/1 -> PID_Parameter/1
  Constant4/1 -> Unit Delay/1
  Unit Delay/1 -> Speak/Enable

== system et_robocon_dev_guy/Main Controller/normal_operation_modes.line_tracking_mode/line_tracking_mode.processLight/LineTracePID/SwitchController/BasicStage/CenterStraight ==
  EC_reseted : Inport
  BasicFwd : Inport  Port=2
  PID_Param : Inport  Port=3
  Enable : EnablePort
  Constant4 : Constant  Value=0
  Normal : Subsystem  TreatAsAtomicUnit=on
  Speak : Subsystem  TreatAsAtomicUnit=on
  Terminator : Terminator
  Unit Delay : UnitDelay  InitialCondition=1  SampleTime=-1
  PID_Parameter : Outport
  fwd : Outport  Port=2
  bias : Outport  Port=3
  wires:
  EC_reseted/1 -> Terminator/1
  Normal/1(Out1) -> bias/1
  PID_Param/1 -> PID_Parameter/1
  BasicFwd/1 -> Normal/1(Fwd)
  Normal/2(fwd) -> fwd/1
  Constant4/1 -> Unit Delay/1
  Unit Delay/1 -> Speak/Enable

== system et_robocon_dev_guy/Main Controller/normal_operation_modes.line_tracking_mode/line_tracking_mode.processLight/LineTracePID/SwitchController/BasicStage/LastStraight ==
  EC_reseted : Inport
  BasicFwd : Inport  Port=2
  PID_Param : Inport  Port=3
  Enable : EnablePort
  Normal : Subsystem  TreatAsAtomicUnit=on
  Terminator : Terminator
  PID_Parameter : Outport
  fwd : Outport  Port=2
  bias : Outport  Port=3
  wires:
  EC_reseted/1 -> Terminator/1
  Normal/1(Out1) -> bias/1
  PID_Param/1 -> PID_Parameter/1
  BasicFwd/1 -> Normal/1(Fwd)
  Normal/2(fwd) -> fwd/1

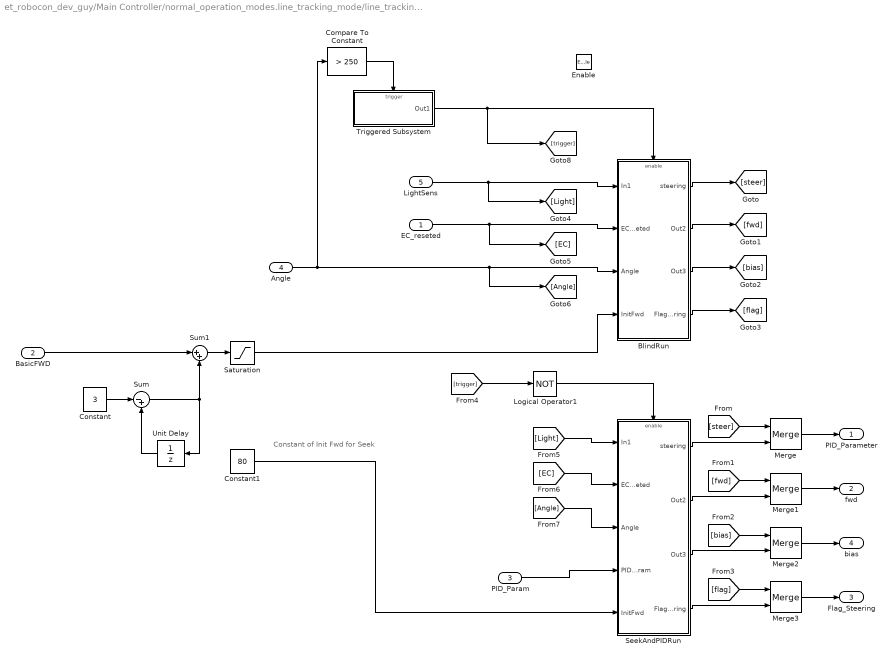
== system et_robocon_dev_guy/Main Controller/normal_operation_modes.line_tracking_mode/line_tracking_mode.processLight/LineTracePID/SwitchController/BasicStage/ShortCut ==
  note: Constant of Init Fwd for Seek
  EC_reseted : Inport
  BasicFWD : Inport  Port=2
  PID_Param : Inport  Port=3
  Angle : Inport  Port=4
  LightSens : Inport  Port=5
  Enable : EnablePort
  BlindRun : Subsystem
  Compare To Constant : simulink/Logic and Bit Operations/Compare To Constant  relop=>  const=250  OutDataTypeStr=boolean
  Constant : Constant  Value=3  OutDataTypeStr=single
  Constant1 : Constant  Value=80  OutDataTypeStr=single
  Logical Operator1 : Logic  Operator=NOT  AllPortsSameDT=off  OutDataTypeStr=boolean
  Merge{,1..3} (4 alike) : Merge
  Saturation : Saturate  UpperLimit=140  LowerLimit=80
  SeekAndPIDRun : Subsystem
  Sum : Sum  Inputs=|-+
  Sum1 : Sum  Inputs=|++
  Triggered Subsystem : Subsystem  TreatAsAtomicUnit=on
  Unit Delay : UnitDelay  SampleTime=-1
  PID_Parameter : Outport
  fwd : Outport  Port=2
  Flag_Steering : Outport  Port=3
  bias : Outport  Port=4
  wires:
  LightSens/1 -> [Light], BlindRun/1(In1)
  EC_reseted/1 -> [EC], BlindRun/2(EC_reseted)
  Merge3/1 -> Flag_Steering/1
  Merge2/1 -> bias/1
  Merge1/1 -> fwd/1
  Merge/1 -> PID_Parameter/1
  SeekAndPIDRun/1(steering) -> Merge/2
  SeekAndPIDRun/2(Out2) -> Merge1/2
  SeekAndPIDRun/3(Out3) -> Merge2/2
  SeekAndPIDRun/4(Flag_Steering) -> Merge3/2
  Compare To Constant/1 -> Triggered Subsystem/Trigger
  Triggered Subsystem/1(Out1) -> BlindRun/Enable, [trigger]
  Angle/1 -> Compare To Constant/1, [Angle], BlindRun/3(Angle)
  PID_Param/1 -> SeekAndPIDRun/4(PID_Param)
  BlindRun/1(steering) -> [steer]
  BlindRun/2(Out2) -> [fwd]
  BlindRun/3(Out3) -> [bias]
  BlindRun/4(Flag_Steering) -> [flag]
  [flag] -> Merge3/1
  [bias] -> Merge2/1
  [fwd] -> Merge1/1
  [steer] -> Merge/1
  Logical Operator1/1 -> SeekAndPIDRun/Enable
  [trigger] -> Logical Operator1/1
  [Light] -> SeekAndPIDRun/1(In1)
  [EC] -> SeekAndPIDRun/2(EC_reseted)
  [Angle] -> SeekAndPIDRun/3(Angle)
  BasicFWD/1 -> Sum1/1
  Sum1/1 -> Saturation/1
  Sum/1 -> Unit Delay/1, Sum1/2
  Unit Delay/1 -> Sum/2
  Constant/1 -> Sum/1
  Saturation/1 -> BlindRun/4(InitFwd)
  Constant1/1 -> SeekAndPIDRun/5(InitFwd)

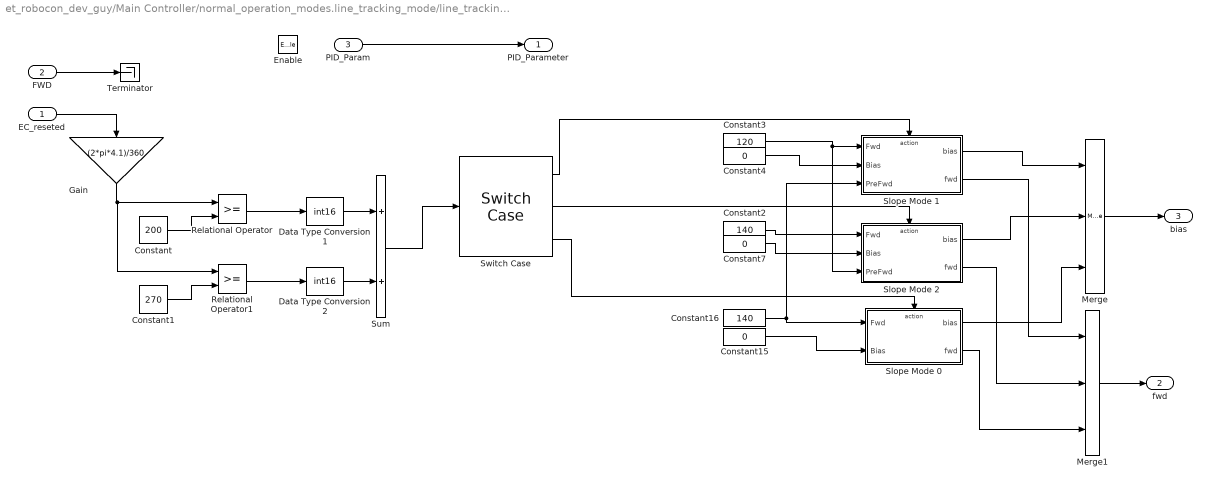
== system et_robocon_dev_guy/Main Controller/normal_operation_modes.line_tracking_mode/line_tracking_mode.processLight/LineTracePID/SwitchController/BasicStage/Slope ==
  EC_reseted : Inport
  FWD : Inport  Port=2
  PID_Param : Inport  Port=3
  Enable : EnablePort
  Constant : Constant  Value=200  OutDataTypeStr=single
  Constant1 : Constant  Value=270  OutDataTypeStr=single
  Constant15 : Constant  Value=0  OutDataTypeStr=single  SampleTime=-1
  Constant16 : Constant  Value=140  OutDataTypeStr=single  SampleTime=-1
  Constant2 : Constant  Value=140  OutDataTypeStr=single  SampleTime=-1
  Constant3 : Constant  Value=120  OutDataTypeStr=single  SampleTime=-1
  Constant4 : Constant  Value=0  OutDataTypeStr=single  SampleTime=-1
  Constant7 : Constant  Value=0  OutDataTypeStr=single  SampleTime=-1
  Data Type Conversion1 : DataTypeConversion  OutDataTypeStr=int16
  Data Type Conversion2 : DataTypeConversion  OutDataTypeStr=int16
  Gain : Gain  Gain=(2*pi*4.1)/360
  Merge : Merge  Inputs=3
  Merge1 : Merge  Inputs=3
  Relational Operator : RelationalOperator  OutDataTypeStr=boolean
  Relational Operator1 : RelationalOperator  OutDataTypeStr=boolean
  Slope Mode 0 : Subsystem  TreatAsAtomicUnit=on
  Slope Mode 1 : Subsystem  TreatAsAtomicUnit=on
  Slope Mode 2 : Subsystem  TreatAsAtomicUnit=on
  Sum : Sum
  Switch Case : SwitchCase  CaseConditions={1,2}
  Terminator : Terminator
  PID_Parameter : Outport
  fwd : Outport  Port=2
  bias : Outport  Port=3
  wires:
  PID_Param/1 -> PID_Parameter/1
  EC_reseted/1 -> Gain/1
  Constant/1 -> Relational Operator/2
  Constant1/1 -> Relational Operator1/2
  Relational Operator/1 -> Data Type Conversion1/1
  Sum/1 -> Switch Case/1
  Relational Operator1/1 -> Data Type Conversion2/1
  Gain/1 -> Relational Operator/1, Relational Operator1/1
  Data Type Conversion1/1 -> Sum/1
  Data Type Conversion2/1 -> Sum/2
  Constant3/1 -> Slope Mode 2/3(PreFwd), Slope Mode 1/1(Fwd)
  Constant4/1 -> Slope Mode 1/2(Bias)
  Switch Case/1 -> Slope Mode 1/Action
  Constant7/1 -> Slope Mode 2/2(Bias)
  Switch Case/2 -> Slope Mode 2/Action
  Constant15/1 -> Slope Mode 0/2(Bias)
  Constant16/1 -> Slope Mode 1/3(PreFwd), Slope Mode 0/1(Fwd)
  Switch Case/3 -> Slope Mode 0/Action
  Slope Mode 1/1(bias) -> Merge/1
  Slope Mode 2/1(bias) -> Merge/2
  Slope Mode 1/2(fwd) -> Merge1/1
  Slope Mode 2/2(fwd) -> Merge1/2
  Merge1/1 -> fwd/1
  Merge/1 -> bias/1
  Constant2/1 -> Slope Mode 2/1(Fwd)
  FWD/1 -> Terminator/1
  Slope Mode 0/2(fwd) -> Merge1/3
  Slope Mode 0/1(bias) -> Merge/3

== system et_robocon_dev_guy/Main Controller/normal_operation_modes.line_tracking_mode/line_tracking_mode.processLight/LineTracePID/SwitchController/BonusStage/Gate ==
  EC_reseted : Inport
  BasicFwd : Inport  Port=2
  Gyro : Inport  Port=3
  LightSens : Inport  Port=4
  PID_Param : Inport  Port=5
  Enable : EnablePort
  Constant2 : Constant  Value=0  OutDataTypeStr=single  SampleTime=-1
  Normal : Subsystem  TreatAsAtomicUnit=on
  SlowDown : Subsystem
  Terminator : Terminator
  Terminator1 : Terminator
  Terminator2 : Terminator
  PID_Parameter : Outport
  fwd : Outport  Port=2
  bias : Outport  Port=3
  wires:
  Normal/2(fwd) -> fwd/1
  Normal/1(Out1) -> bias/1
  PID_Param/1 -> PID_Parameter/1
  EC_reseted/1 -> Terminator1/1
  Gyro/1 -> Terminator2/1
  LightSens/1 -> Terminator/1
  Constant2/1 -> SlowDown/1(TargetFwd)
  BasicFwd/1 -> SlowDown/2(LastFwd)
  SlowDown/1(fwd) -> Normal/1(Fwd)

== system et_robocon_dev_guy/Main Controller/normal_operation_modes.line_tracking_mode/line_tracking_mode.processLight/LineTracePID/SwitchController/BonusStage/IntoGarage ==
  EC_reseted : Inport
  BasicFwd : Inport  Port=2
  Gyro : Inport  Port=3
  LightSens : Inport  Port=4
  PID_Param : Inport  Port=5
  Enable : EnablePort
  Normal : Subsystem  TreatAsAtomicUnit=on
  Terminator : Terminator
  Terminator1 : Terminator
  Terminator2 : Terminator
  PID_Parameter : Outport
  fwd : Outport  Port=2
  bias : Outport  Port=3
  wires:
  LightSens/1 -> Terminator/1
  Gyro/1 -> Terminator2/1
  EC_reseted/1 -> Terminator1/1
  PID_Param/1 -> PID_Parameter/1
  Normal/1(Out1) -> bias/1
  Normal/2(fwd) -> fwd/1
  BasicFwd/1 -> Normal/1(Fwd)

== system et_robocon_dev_guy/Main Controller/normal_operation_modes.line_tracking_mode/line_tracking_mode.processLight/LineTracePID/SwutchForFreeSteering/tmpController/Derivative ==
  In : Inport
  Constant2 : Constant  Value=Ts_  OutDataTypeStr=single  SampleTime=-1
  Difference : simulink/Discrete/Difference  ICPrevInput=0.0  InputProcessing=Inherited  OutMin=[]  OutMax=[]  OutDataTypeStr=single  OutputDataTypeScalingMode=single  OutDataType=sfix(16)  OutScaling=2^-10  RndMeth=Nearest  DoSatur=off
  Divide4 : Product  Inputs=*/  OutDataTypeStr=single  RndMeth=Nearest
  Out : Outport
  wires:
  Constant2/1 -> Divide4/2
  Divide4/1 -> Difference/1
  In/1 -> Divide4/1
  Difference/1 -> Out/1

== system et_robocon_dev_guy/Main Controller/normal_operation_modes.line_tracking_mode/line_tracking_mode.processLight/LineTracePID/SwutchForFreeSteering/tmpController/Fillter ==
  In : Inport
  In1 : Inport  Port=2
  Add : Sum  RndMeth=Nearest
  Add2 : Sum  Inputs=+-  OutDataTypeStr=single  RndMeth=Nearest
  Constant : Constant  Value=single(1-(0.0001/(0.1*Ts_)))  OutDataTypeStr=single  SampleTime=-1
  Constant1 : Constant  Value=single(0.0001/(0.1*Ts_))  OutDataTypeStr=single  SampleTime=-1
  Constant2 : Constant  Value=(0.1*Ts_)  OutDataTypeStr=single  SampleTime=-1
  Constant3 : Constant  OutDataTypeStr=single  SampleTime=-1
  Constant4 : Constant  Value=0.00001  OutDataTypeStr=single  SampleTime=-1
  Constant6 : Constant  Value=(0.1*Ts_)  OutDataTypeStr=single  SampleTime=-1
  Divide : Product  Inputs=*/
  Divide1 : Product  Inputs=*/
  Manual Switch1 : ManualSwitch  CurrentSetting=0
  Manual Switch3 : ManualSwitch  CurrentSetting=0
  Product : Product  OutDataTypeStr=single  RndMeth=Nearest
  Product1 : Product  OutDataTypeStr=single  RndMeth=Nearest
  Product3 : Product  OutDataTypeStr=single  RndMeth=Nearest
  Unit Delay : UnitDelay  SampleTime=-1
  Unit Delay1 : UnitDelay  SampleTime=-1
  Out : Outport
  wires:
  In/1 -> Unit Delay1/1
  Unit Delay1/1 -> Product1/1
  Product1/1 -> Add/1
  Unit Delay/1 -> Product/2
  Add/1 -> Out/1, Unit Delay/1
  Product/1 -> Add/2
  Constant6/1 -> Divide/2
  Constant2/1 -> Divide1/2
  Divide1/1 -> Add2/2
  In1/1 -> Product3/1
  Product3/1 -> Divide1/1, Divide/1
  Constant4/1 -> Product3/2
  Constant3/1 -> Add2/1
  Manual Switch1/1 -> Product1/2
  Constant1/1 -> Manual Switch1/1
  Divide/1 -> Manual Switch1/2
  Manual Switch3/1 -> Product/1
  Constant/1 -> Manual Switch3/1
  Add2/1 -> Manual Switch3/2

== system et_robocon_dev_guy/Main Controller/normal_operation_modes.line_tracking_mode/line_tracking_mode.processLight/LineTracePID/SwutchForFreeSteering/tmpController/I_over_guard ==
  In1 : Inport
  Compare To Constant1 : simulink/Logic and Bit Operations/Compare To Constant  relop===  const=1  OutDataTypeStr=uint8
  Constant2 : Constant  Value=0  OutDataTypeStr=uint8  SampleTime=-1
  Constant4 : Constant  Value=0  OutDataTypeStr=uint8  SampleTime=-1
  Memory1 : Memory  X0=1  InheritSampleTime=on
  Switch : Switch  Threshold=1
  Out1 : Outport
  wires:
  Memory1/1 -> Compare To Constant1/1
  Constant2/1 -> Memory1/1
  Constant4/1 -> Switch/1
  Compare To Constant1/1 -> Switch/2
  Switch/1 -> Out1/1
  In1/1 -> Switch/3

== system et_robocon_dev_guy/Main Controller/normal_operation_modes.line_tracking_mode/line_tracking_mode.processLight/LineTracePID/SwutchForFreeSteering/tmpController/Integrator ==
  In : Inport
  Constant2 : Constant  Value=Ts_  OutDataTypeStr=single  SampleTime=-1
  Integrator : DiscreteTransferFcn  Denominator=[1 -1]  RndMeth=Nearest
  Product1 : Product  OutDataTypeStr=single  RndMeth=Nearest
  Out : Outport
  wires:
  Constant2/1 -> Product1/2
  Product1/1 -> Integrator/1
  In/1 -> Product1/1
  Integrator/1 -> Out/1

== system et_robocon_dev_guy/Main Controller/normal_operation_modes.line_tracking_mode/line_tracking_mode.processLight/LineTracePID/SwitchController/BasicStage/4thCorner/Normal ==
  Fwd : Inport
  Constant2 : Constant  Value=-10  OutDataTypeStr=single  SampleTime=-1
  Out1 : Outport
  fwd : Outport  Port=2
  wires:
  Constant2/1 -> Out1/1
  Fwd/1 -> fwd/1

== system et_robocon_dev_guy/Main Controller/normal_operation_modes.line_tracking_mode/line_tracking_mode.processLight/LineTracePID/SwitchController/BasicStage/4thCorner/SlowDown ==
  TargetFwd : Inport
  LastFwd : Inport  Port=2
  Constant1 : Constant  Value=-4  OutDataTypeStr=single  SampleTime=-1
  Saturation1 : Saturate  UpperLimit=160  LowerLimit=80  RndMeth=Simplest
  Sum1 : Sum  Inputs=+-  AccumDataTypeStr=single  OutDataTypeStr=single  RndMeth=Simplest
  Sum2 : Sum  Inputs=|++  AccumDataTypeStr=single  OutDataTypeStr=single  RndMeth=Simplest  InputSameDT=on
  Sum3 : Sum  Inputs=|++  AccumDataTypeStr=single  OutDataTypeStr=single  RndMeth=Simplest  InputSameDT=on
  Switch : Switch  Criteria=u2 > Threshold  OutDataTypeStr=single  RndMeth=Simplest
  Unit Delay1 : UnitDelay  SampleTime=-1
  fwd : Outport
  wires:
  TargetFwd/1 -> Switch/1, Sum1/1
  Switch/1 -> fwd/1
  Sum1/1 -> Switch/2
  Unit Delay1/1 -> Sum2/2
  LastFwd/1 -> Sum3/1
  Constant1/1 -> Sum2/1
  Sum3/1 -> Saturation1/1
  Saturation1/1 -> Switch/3, Sum1/2
  Sum2/1 -> Sum3/2, Unit Delay1/1

== system et_robocon_dev_guy/Main Controller/normal_operation_modes.line_tracking_mode/line_tracking_mode.processLight/LineTracePID/SwitchController/BasicStage/4thCorner/Speak ==
  Enable : EnablePort
  Constant : Constant  Value=50
  Speaker : legonxtlib/Speaker  sinputMode=Volume only  sspeakerFreq=800  sspeakerVolume=50  sspeakerDuration=100
  wires:
  Constant/1 -> Speaker/1

== system et_robocon_dev_guy/Main Controller/normal_operation_modes.line_tracking_mode/line_tracking_mode.processLight/LineTracePID/SwitchController/BasicStage/5thCorner/Normal ==
  Fwd : Inport
  Constant2 : Constant  Value=-10  OutDataTypeStr=single  SampleTime=-1
  Out1 : Outport
  fwd : Outport  Port=2
  wires:
  Fwd/1 -> fwd/1
  Constant2/1 -> Out1/1

== system et_robocon_dev_guy/Main Controller/normal_operation_modes.line_tracking_mode/line_tracking_mode.processLight/LineTracePID/SwitchController/BasicStage/5thCorner/SlowDown ==
  TargetFwd : Inport
  LastFwd : Inport  Port=2
  Constant1 : Constant  Value=-4  OutDataTypeStr=single  SampleTime=-1
  Saturation1 : Saturate  UpperLimit=160  LowerLimit=80  RndMeth=Simplest
  Sum1 : Sum  Inputs=+-  AccumDataTypeStr=single  OutDataTypeStr=single  RndMeth=Simplest
  Sum2 : Sum  Inputs=|++  AccumDataTypeStr=single  OutDataTypeStr=single  RndMeth=Simplest  InputSameDT=on
  Sum3 : Sum  Inputs=|++  AccumDataTypeStr=single  OutDataTypeStr=single  RndMeth=Simplest  InputSameDT=on
  Switch : Switch  Criteria=u2 > Threshold  OutDataTypeStr=single  RndMeth=Simplest
  Unit Delay1 : UnitDelay  SampleTime=-1
  fwd : Outport
  wires:
  TargetFwd/1 -> Switch/1, Sum1/1
  Switch/1 -> fwd/1
  Sum1/1 -> Switch/2
  Unit Delay1/1 -> Sum2/2
  LastFwd/1 -> Sum3/1
  Constant1/1 -> Sum2/1
  Sum3/1 -> Saturation1/1
  Saturation1/1 -> Switch/3, Sum1/2
  Sum2/1 -> Sum3/2, Unit Delay1/1

== system et_robocon_dev_guy/Main Controller/normal_operation_modes.line_tracking_mode/line_tracking_mode.processLight/LineTracePID/SwitchController/BasicStage/5thCorner/Speak ==
  Enable : EnablePort
  Constant : Constant  Value=50
  Speaker : legonxtlib/Speaker  sinputMode=Volume only  sspeakerFreq=800  sspeakerVolume=50  sspeakerDuration=100
  wires:
  Constant/1 -> Speaker/1

== system et_robocon_dev_guy/Main Controller/normal_operation_modes.line_tracking_mode/line_tracking_mode.processLight/LineTracePID/SwitchController/BasicStage/6thCorner/Normal ==
  Fwd : Inport
  Constant2 : Constant  Value=10  OutDataTypeStr=single  SampleTime=-1
  Out1 : Outport
  fwd : Outport  Port=2
  wires:
  Constant2/1 -> Out1/1
  Fwd/1 -> fwd/1

== system et_robocon_dev_guy/Main Controller/normal_operation_modes.line_tracking_mode/line_tracking_mode.processLight/LineTracePID/SwitchController/BasicStage/6thCorner/Speak ==
  Enable : EnablePort
  Constant : Constant  Value=50
  Speaker : legonxtlib/Speaker  sinputMode=Volume only  sspeakerFreq=800  sspeakerVolume=50  sspeakerDuration=100
  wires:
  Constant/1 -> Speaker/1
